simulink model "Thermal_model_of_a_house"  (R2025b)
settings: Solver=VariableStepAuto  StartTime=0.0  StopTime=24  RelTol=1e-3
undefined symbols (not defined in the file): c, Ce, m, mdot, R_th, Tavg, Th, Ts
settings Model: Creator=Samuel  LastModifiedBy=Samuel

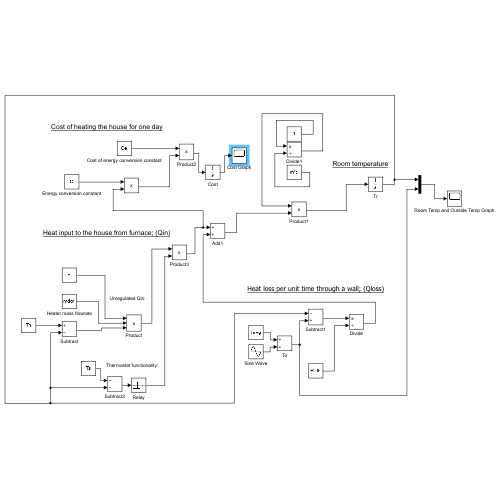
[thumbnail: Simulink's stored preview of the top-level diagram]
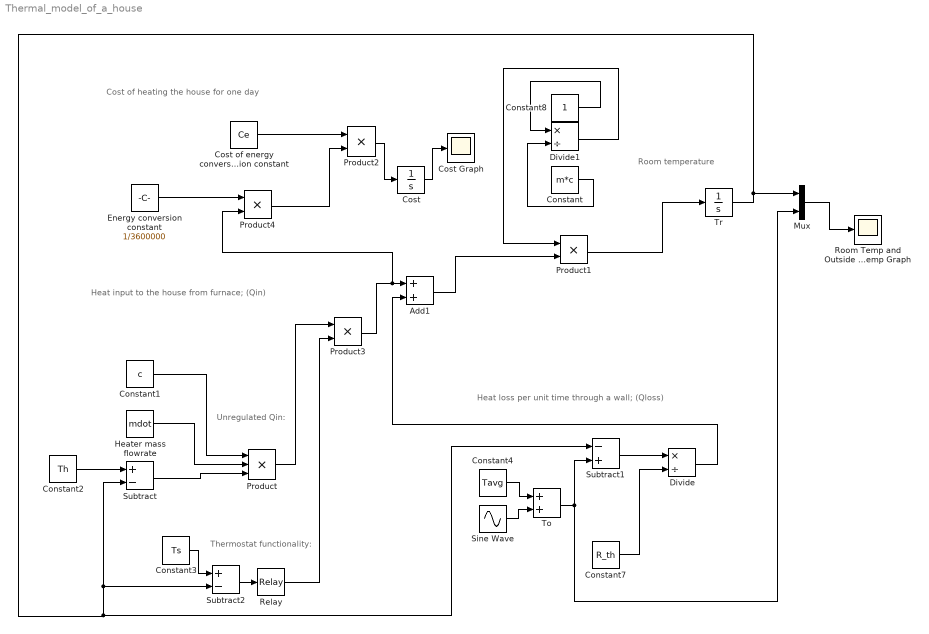
== system Thermal_model_of_a_house ==
  note: Cost of heating the house for one day
  note: Unregulated Qin:
  note: Thermostat functionality:
  note: Room temperature
  note: Heat loss per unit time through a wall; (Qloss)
  note: Heat input to the house from furnace; (Qin)
  Add1 : Sum
  Constant : Constant  Value=m*c
  Constant1 : Constant  Value=c
  Constant2 : Constant  Value=Th
  Constant3 : Constant  Value=Ts
  Constant4 : Constant  Value=Tavg
  Constant7 : Constant  Value=R_th
  Constant8 : Constant
  Cost : Integrator
  Cost Graph : Scope
      settings: ActiveDisplayYMinimum=-1.2975835075184745  ActiveDisplayYMaximum=11.678251567666273
  Cost of energy conversion constant : Constant  Value=Ce
  Divide : Product  Inputs=*/
  Divide1 : Product  Inputs=*/
  Energy conversion constant : Constant  Value=1/3600000
  Heater mass flowrate : Constant  Value=mdot
  Mux : Mux  Inputs=2
  Product : Product  Inputs=3
  Product{1..4} (4 alike) : Product
  Relay : Relay  OnSwitchValue=2  OffSwitchValue=-2
  Room Temp and Outside Temp Graph : Scope
      settings: ActiveDisplayYMinimum=5.12500592230363  ActiveDisplayYMaximum=23.874999341973663
  Sine Wave : Sin  Amplitude=5  Frequency=(2*pi)/24  SampleTime=0
  Subtract : Sum  Inputs=+-
  Subtract1 : Sum  Inputs=-+
  Subtract2 : Sum  Inputs=+-
  To : Sum
  Tr : Integrator  InitialCondition=20
  wires:
  Constant1/1 -> Product/1
  Constant2/1 -> Subtract/1
  Subtract/1 -> Product/3
  To/1 -> Mux/2, Subtract1/2
  Constant4/1 -> To/1
  Tr/1 -> Mux/1, Subtract/2, Subtract2/2, Subtract1/1
  Sine Wave/1 -> To/2
  Subtract1/1 -> Divide/1
  Constant7/1 -> Divide/2
  Divide/1 -> Add1/2
  Constant8/1 -> Divide1/1
  Divide1/1 -> Product1/1
  Add1/1 -> Product1/2
  Product1/1 -> Tr/1
  Constant/1 -> Divide1/2
  Subtract2/1 -> Relay/1
  Constant3/1 -> Subtract2/1
  Product3/1 -> Product4/2, Add1/1
  Heater mass flowrate/1 -> Product/2
  Product/1 -> Product3/1
  Relay/1 -> Product3/2
  Mux/1 -> Room Temp and Outside Temp Graph/1
  Cost of energy conversion constant/1 -> Product2/1
  Energy conversion constant/1 -> Product4/1
  Product4/1 -> Product2/2
  Product2/1 -> Cost/1
  Cost/1 -> Cost Graph/1
